simulink model "AircraftModel_6DoF"  (R2020b)
settings: Solver=VariableStepAuto  StartTime=0.0  StopTime=20  FixedStep=CNT_StepSize  RelTol=1e-3
values from neighbouring files (symbols this model uses):
  CNT_a = 6378137    [AircraftParameters.m]
  CNT_f = 0.003352810664747    (= 0.00335281066475)    [AircraftParameters.m]
  CNT_g = [0;0;9.81]    [AircraftParameters.m]
  CNT_m = 15917    [AircraftParameters.m]
  Ixx = 105390    [AircraftParameters.m]
  Ixz = 15539    [AircraftParameters.m]
  Iyy = 280790    [AircraftParameters.m]
  Izz = 350200    [AircraftParameters.m]
undefined symbols (not defined in the file or in its folder): Actuators, Aerodynamics, Propulsion, TrimPoint
libraries: vrlib x4
settings Model: Creator=NicolasS  LastModifiedBy=NicolasS

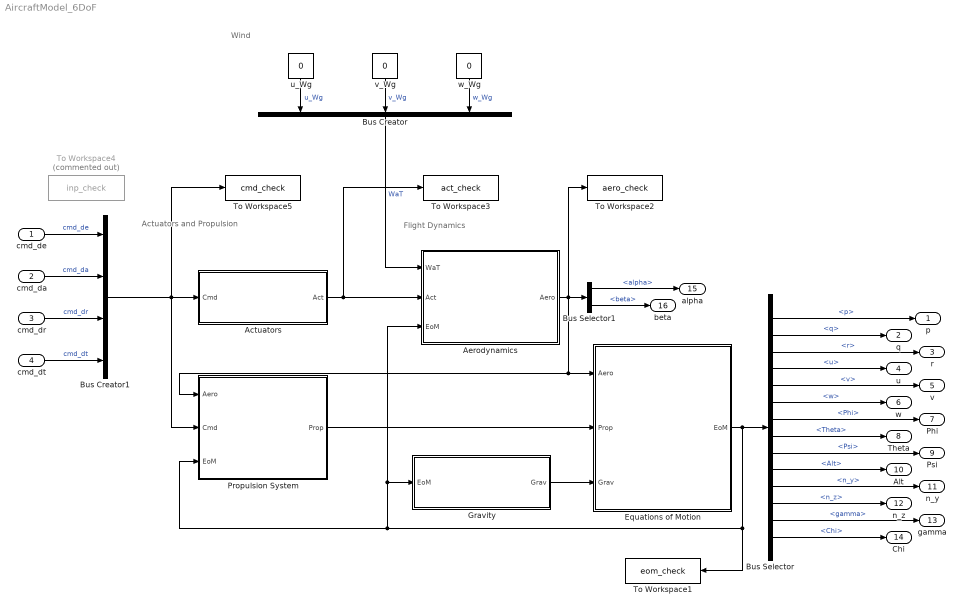
== system AircraftModel_6DoF ==
  note: Wind
  note: Actuators and Propulsion
  note: Flight Dynamics
  cmd_de : Inport
  cmd_da : Inport  Port=2
  cmd_dr : Inport  Port=3
  cmd_dt : Inport  Port=4
  Actuators : Subsystem
  Aerodynamics : Subsystem
  Bus Creator : BusCreator  Inputs=3
  Bus Creator1 : BusCreator  Inputs=4  OutDataTypeStr=Bus: Cmd
  Bus Selector : BusSelector  OutputSignals=OOmega_f.p,OOmega_f.q,OOmega_f.r,vv_f.u,vv_f.v,vv_f.w,PPhi.Phi,PPhi.Theta,PPhi.Psi,Position.Alt,nn_f.n_y,nn_f.n_z,TrackData.gamma,TrackData.Chi
  Bus Selector1 : BusSelector  OutputSignals=AirData.alpha,AirData.beta
  Equations of Motion : Subsystem
  Gravity : Subsystem
  "Propulsion System " : Subsystem
  To Workspace1 : ToWorkspace  VariableName=eom_check  SaveFormat=Timeseries  SampleTime=-1
      settings: Decimation=2
  To Workspace2 : ToWorkspace  VariableName=aero_check  SaveFormat=Timeseries  SampleTime=-1
      settings: Decimation=2
  To Workspace3 : ToWorkspace  VariableName=act_check  SaveFormat=Timeseries  SampleTime=-1
      settings: Decimation=2
  To Workspace4 : ToWorkspace  Commented=on  VariableName=inp_check  SaveFormat=Timeseries  SampleTime=-1
      settings: Decimation=2
  To Workspace5 : ToWorkspace  VariableName=cmd_check  SaveFormat=Timeseries  SampleTime=-1
      settings: Decimation=2
  u_Wg : Constant  Value=0  SampleTime=-1
  v_Wg : Constant  Value=0  SampleTime=-1
  w_Wg : Constant  Value=0  SampleTime=-1
  p : Outport  Unit=rad/s
  q : Outport  Port=2  Unit=rad/s
  r : Outport  Port=3  Unit=rad/s
  u : Outport  Port=4  Unit=m/s
  v : Outport  Port=5  Unit=m/s
  w : Outport  Port=6  Unit=m/s
  Phi : Outport  Port=7  Unit=rad
  Theta : Outport  Port=8  Unit=rad
  Psi : Outport  Port=9  Unit=rad
  Alt : Outport  Port=10  Unit=m
  n_y : Outport  Port=11
  n_z : Outport  Port=12
  gamma : Outport  Port=13  Unit=rad
  Chi : Outport  Port=14  Unit=rad
  alpha : Outport  Port=15
  beta : Outport  Port=16
  wires:
  u_Wg/1 -> Bus Creator/1  "u_Wg"
  Actuators/1(Act) -> To Workspace3/1, Aerodynamics/2(Act)
  Aerodynamics/1(Aero) -> To Workspace2/1, Bus Selector1/1, Equations of Motion/1(Aero), "Propulsion System "/1(Aero)
  w_Wg/1 -> Bus Creator/3  "w_Wg"
  Equations of Motion/1(EoM) -> To Workspace1/1, Aerodynamics/3(EoM), Gravity/1(EoM), "Propulsion System "/3(EoM), Bus Selector/1
  "Propulsion System "/1(Prop) -> Equations of Motion/2(Prop)
  Gravity/1(Grav) -> Equations of Motion/3(Grav)
  Bus Creator/1 -> Aerodynamics/1(WaT)  "WaT"
  Bus Selector1/2 -> beta/1  "<beta>"
  v_Wg/1 -> Bus Creator/2  "v_Wg"
  cmd_de/1 -> Bus Creator1/1  "cmd_de"
  cmd_dr/1 -> Bus Creator1/3  "cmd_dr"
  cmd_da/1 -> Bus Creator1/2  "cmd_da"
  cmd_dt/1 -> Bus Creator1/4  "cmd_dt"
  Bus Selector/3 -> r/1  "<r>"
  Bus Selector/9 -> Psi/1  "<Psi>"
  Bus Selector/7 -> Phi/1  "<Phi>"
  Bus Selector/1 -> p/1  "<p>"
  Bus Selector/11 -> n_y/1  "<n_y>"
  Bus Selector1/1 -> alpha/1  "<alpha>"
  Bus Selector/2 -> q/1  "<q>"
  Bus Selector/6 -> w/1  "<w>"
  Bus Selector/4 -> u/1  "<u>"
  Bus Selector/12 -> n_z/1  "<n_z>"
  Bus Selector/10 -> Alt/1  "<Alt>"
  Bus Selector/8 -> Theta/1  "<Theta>"
  Bus Creator1/1 -> To Workspace5/1, "Propulsion System "/2(Cmd), Actuators/1(Cmd)
  Bus Selector/13 -> gamma/1  "<gamma>"
  Bus Selector/14 -> Chi/1  "<Chi>"
  Bus Selector/5 -> v/1  "<v>"

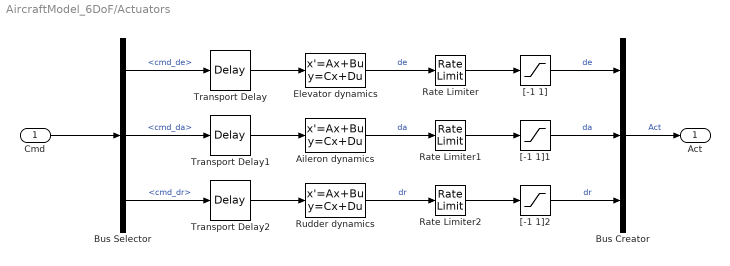
== system AircraftModel_6DoF/Actuators ==
  Cmd : Inport  OutDataTypeStr=Bus: Cmd
  Aileron dynamics : StateSpace  A=Actuators.Act_a.A  B=Actuators.Act_a.B  C=Actuators.Act_a.C  D=Actuators.Act_a.D  InitialCondition=TrimPoint.States.dabar  ContinuousStateAttributes='da'
  Bus Creator : BusCreator  Inputs=3  OutDataTypeStr=Bus: Act
  Bus Selector : BusSelector  OutputSignals=cmd_de,cmd_da,cmd_dr
  Elevator dynamics : StateSpace  A=Actuators.Act_e.A  B=Actuators.Act_e.B  C=Actuators.Act_e.C  D=Actuators.Act_e.D  InitialCondition=TrimPoint.States.debar  ContinuousStateAttributes='de'
  Rate Limiter : RateLimiter  RisingSlewLimit=max(Actuators.RateLimits.udot_max_He)  FallingSlewLimit=min(Actuators.RateLimits.udot_max_He)  SampleTimeMode=inherited
  Rate Limiter1 : RateLimiter  RisingSlewLimit=max(Actuators.RateLimits.udot_max_Ha)  FallingSlewLimit=min(Actuators.RateLimits.udot_max_Ha)  SampleTimeMode=inherited
  Rate Limiter2 : RateLimiter  RisingSlewLimit=max(Actuators.RateLimits.udot_max_Hr)  FallingSlewLimit=min(Actuators.RateLimits.udot_max_Hr)  SampleTimeMode=inherited
  Rudder dynamics : StateSpace  A=Actuators.Act_r.A  B=Actuators.Act_r.B  C=Actuators.Act_r.C  D=Actuators.Act_r.D  InitialCondition=TrimPoint.States.drbar  ContinuousStateAttributes='dr'
  Transport Delay : TransportDelay  DelayTime=Actuators.Delays.tau_de  InitialOutput=TrimPoint.States.debar  TransDelayFeedthrough=on
  Transport Delay1 : TransportDelay  DelayTime=Actuators.Delays.tau_da  InitialOutput=TrimPoint.States.dabar  TransDelayFeedthrough=on
  Transport Delay2 : TransportDelay  DelayTime=Actuators.Delays.tau_dr  InitialOutput=TrimPoint.States.drbar  TransDelayFeedthrough=on
  "[-1 1]" : Saturate  UpperLimit=max(Actuators.Limits.u_max_He)  LowerLimit=min(Actuators.Limits.u_max_He)
  "[-1 1]1" : Saturate  UpperLimit=max(Actuators.Limits.u_max_Ha)  LowerLimit=min(Actuators.Limits.u_max_Ha)
  "[-1 1]2" : Saturate  UpperLimit=max(Actuators.Limits.u_max_Hr)  LowerLimit=min(Actuators.Limits.u_max_Hr)
  Act : Outport  OutDataTypeStr=Bus: Act
  wires:
  Elevator dynamics/1 -> Rate Limiter/1  "de"
  "[-1 1]1"/1 -> Bus Creator/2  "da"
  Rudder dynamics/1 -> Rate Limiter2/1  "dr"
  Transport Delay1/1 -> Aileron dynamics/1
  Cmd/1 -> Bus Selector/1
  "[-1 1]"/1 -> Bus Creator/1  "de"
  Bus Selector/1 -> Transport Delay/1  "<cmd_de>"
  Transport Delay/1 -> Elevator dynamics/1
  "[-1 1]2"/1 -> Bus Creator/3  "dr"
  Transport Delay2/1 -> Rudder dynamics/1
  Aileron dynamics/1 -> Rate Limiter1/1  "da"
  Bus Selector/3 -> Transport Delay2/1  "<cmd_dr>"
  Bus Creator/1 -> Act/1  "Act"
  Bus Selector/2 -> Transport Delay1/1  "<cmd_da>"
  Rate Limiter/1 -> "[-1 1]"/1
  Rate Limiter1/1 -> "[-1 1]1"/1
  Rate Limiter2/1 -> "[-1 1]2"/1

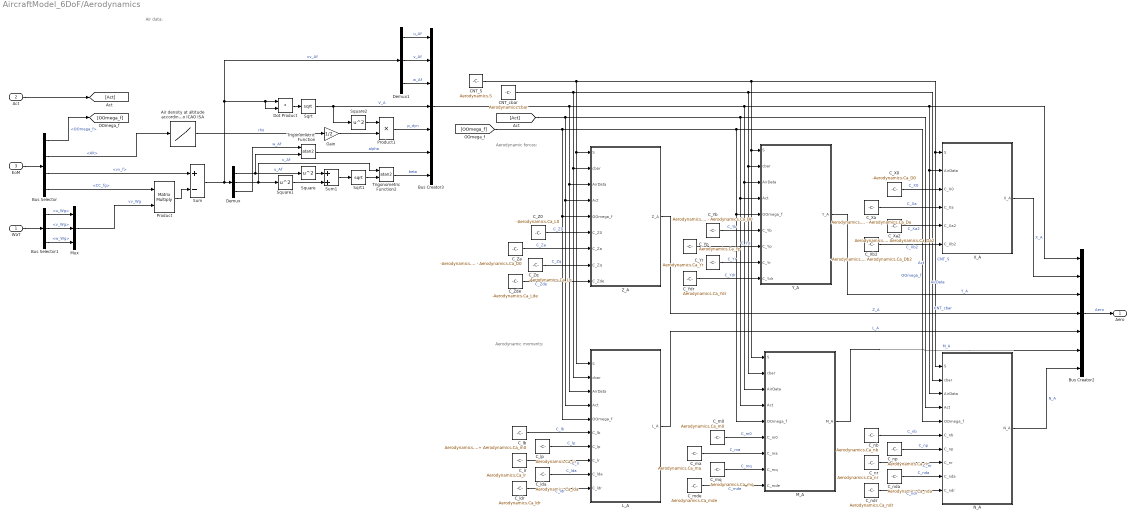
== system AircraftModel_6DoF/Aerodynamics ==
  note: Air data:
  note: Aerodynamic moments:
  note: Aerodynamic forces:
  WaT : Inport  OutDataTypeStr=Bus: WaT
  Act : Inport  Port=2  OutDataTypeStr=Bus: Act
  EoM : Inport  Port=3  OutDataTypeStr=Bus: EoM
  Air density at altitude according to ICAO ISA : Lookup_n-D  NumberOfTableDimensions=1  BreakpointsForDimension1=Aerodynamics.LUT_Alt  Table=Aerodynamics.LUT_rho  ExtrapMethod=Clip  InternalRulePriority=Speed  RndMeth=Simplest  InputSameDT=on
  Bus Creator2 : BusCreator  Inputs=7  OutDataTypeStr=Bus: Aero
  Bus Creator3 : BusCreator  Inputs=7  OutDataTypeStr=Bus: AirData
  Bus Selector : BusSelector  OutputSignals=OOmega_f,Position.Alt,vv_f,CC.CC_fg
  Bus Selector1 : BusSelector  OutputSignals=u_Wg,v_Wg,w_Wg
  CNT_S : Constant  Value=Aerodynamics.S  OutDataTypeStr=double  SampleTime=-1
  CNT_cbar : Constant  Value=Aerodynamics.cbar  OutDataTypeStr=double  SampleTime=-1
  C_X0 : Constant  Value=-Aerodynamics.Ca_D0  VectorParams1D=off  OutDataTypeStr=double  SampleTime=-1
  C_Xa : Constant  Value=Aerodynamics.Ca_L0 - Aerodynamics.Ca_Da  VectorParams1D=off  OutDataTypeStr=double  SampleTime=-1
  C_Xa2 : Constant  Value=Aerodynamics.Ca_La - Aerodynamics.Ca_Da2  VectorParams1D=off  OutDataTypeStr=double  SampleTime=-1
  C_Xb2 : Constant  Value=-Aerodynamics.Ca_Yb - Aerodynamics.Ca_Db2  VectorParams1D=off  OutDataTypeStr=double  SampleTime=-1
  C_Yb : Constant  Value=Aerodynamics.Ca_Yb - Aerodynamics.Ca_D0  VectorParams1D=off  OutDataTypeStr=double  SampleTime=-1
  C_Ydr : Constant  Value=Aerodynamics.Ca_Ydr  VectorParams1D=off  OutDataTypeStr=double  SampleTime=-1
  C_Yp : Constant  Value=Aerodynamics.Ca_Yp  VectorParams1D=off  OutDataTypeStr=double  SampleTime=-1
  C_Yr : Constant  Value=Aerodynamics.Ca_Yr  VectorParams1D=off  OutDataTypeStr=double  SampleTime=-1
  C_Z0 : Constant  Value=-Aerodynamics.Ca_L0  VectorParams1D=off  OutDataTypeStr=double  SampleTime=-1
  C_Za : Constant  Value=-Aerodynamics.Ca_La - Aerodynamics.Ca_D0  VectorParams1D=off  OutDataTypeStr=double  SampleTime=-1
  C_Zde : Constant  Value=-Aerodynamics.Ca_Lde  VectorParams1D=off  OutDataTypeStr=double  SampleTime=-1
  C_Zq : Constant  Value=-Aerodynamics.Ca_Lq  VectorParams1D=off  OutDataTypeStr=double  SampleTime=-1
  C_lb : Constant  Value=Aerodynamics.Ca_lb + Aerodynamics.Ca_m0  VectorParams1D=off  OutDataTypeStr=double  SampleTime=-1
  C_lda : Constant  Value=Aerodynamics.Ca_lda  VectorParams1D=off  OutDataTypeStr=double  SampleTime=-1
  C_ldr : Constant  Value=Aerodynamics.Ca_ldr  VectorParams1D=off  OutDataTypeStr=double  SampleTime=-1
  C_lp : Constant  Value=Aerodynamics.Ca_lp  VectorParams1D=off  OutDataTypeStr=double  SampleTime=-1
  C_lr : Constant  Value=Aerodynamics.Ca_lr  VectorParams1D=off  OutDataTypeStr=double  SampleTime=-1
  C_m0 : Constant  Value=Aerodynamics.Ca_m0  VectorParams1D=off  OutDataTypeStr=double  SampleTime=-1
  C_ma : Constant  Value=Aerodynamics.Ca_ma  VectorParams1D=off  OutDataTypeStr=double  SampleTime=-1
  C_mde : Constant  Value=Aerodynamics.Ca_mde  VectorParams1D=off  OutDataTypeStr=double  SampleTime=-1
  C_mq : Constant  Value=Aerodynamics.Ca_mq  VectorParams1D=off  OutDataTypeStr=double  SampleTime=-1
  C_nb : Constant  Value=Aerodynamics.Ca_nb  VectorParams1D=off  OutDataTypeStr=double  SampleTime=-1
  C_nda : Constant  Value=Aerodynamics.Ca_nda  VectorParams1D=off  OutDataTypeStr=double  SampleTime=-1
  C_ndr : Constant  Value=Aerodynamics.Ca_ndr  VectorParams1D=off  OutDataTypeStr=double  SampleTime=-1
  C_np : Constant  Value=Aerodynamics.Ca_np  VectorParams1D=off  OutDataTypeStr=double  SampleTime=-1
  C_nr : Constant  Value=Aerodynamics.Ca_nr  VectorParams1D=off  OutDataTypeStr=double  SampleTime=-1
  Demux : Demux  Outputs=3
  Demux1 : Demux  Outputs=3
  Dot Product : DotProduct  InputSameDT=on  OutDataTypeStr=Inherit: Inherit via internal rule
  Gain : Gain  Gain=1/2
  L_A : MATLAB Function  TreatAsAtomicUnit=on
  M_A : MATLAB Function  TreatAsAtomicUnit=on
  Mux : Mux  Inputs=3
  N_A : MATLAB Function  TreatAsAtomicUnit=on
  Product : Product  Multiplication=Matrix(*)
  Product1 : Product
  Sqrt : Sqrt  SaturateOnIntegerOverflow=on
  Sqrt1 : Sqrt  SaturateOnIntegerOverflow=on
  Square : Math  Operator=square  SaturateOnIntegerOverflow=on
  Square1 : Math  Operator=square  SaturateOnIntegerOverflow=on
  Square2 : Math  Operator=square  SaturateOnIntegerOverflow=on
  Sum : Sum  Inputs=+-
  Sum1 : Sum
  Trigonometric Function : Trigonometry  Operator=atan2
  Trigonometric Function2 : Trigonometry  Operator=atan2
  X_A : MATLAB Function  TreatAsAtomicUnit=on
  Y_A : MATLAB Function  TreatAsAtomicUnit=on
  Z_A : MATLAB Function  TreatAsAtomicUnit=on
  Aero : Outport  OutDataTypeStr=Bus: Aero
  wires:
  Demux1/3 -> Bus Creator3/3  "w_Af"
  C_lp/1 -> L_A/7(C_lp)  "C_lp"
  Act/1 -> [Act]
  N_A/1(N_A) -> Bus Creator2/7  "N_A"
  C_nb/1 -> N_A/6(C_nb)  "C_nb"
  C_ldr/1 -> L_A/10(C_ldr)  "C_ldr"
  C_m0/1 -> M_A/6(C_m0)  "C_m0"
  C_Zq/1 -> Z_A/8(C_Zq)  "C_Zq"
  [OOmega_f] -> N_A/5(OOmega_f), M_A/5(OOmega_f), Y_A/5(OOmega_f), L_A/5(OOmega_f), Z_A/5(OOmega_f)  "OOmega_f"
  C_lr/1 -> L_A/8(C_lr)  "C_lr"
  C_mq/1 -> M_A/8(C_mq)  "C_mq"
  Air density at altitude according to ICAO ISA/1 -> Gain/1  "rho"
  C_Z0/1 -> Z_A/6(C_Z0)  "C_Z0"
  Square/1 -> Sum1/1
  X_A/1(X_A) -> Bus Creator2/2  "X_A"
  Trigonometric Function2/1 -> Bus Creator3/7  "beta"
  C_Yr/1 -> Y_A/8(C_Yr)  "C_Yr"
  C_Yb/1 -> Y_A/6(C_Yb)  "C_Yb"
  Demux1/2 -> Bus Creator3/2  "v_Af"
  Dot Product/1 -> Sqrt/1
  C_ma/1 -> M_A/7(C_ma)  "C_ma"
  C_nda/1 -> N_A/9(C_nda)  "C_nda"
  C_Xa/1 -> X_A/4(C_Xa)  "C_Xa"
  C_lb/1 -> L_A/6(C_lb)  "C_lb"
  Sum/1 -> Demux/1, Demux1/1, Dot Product/2, Dot Product/1  "vv_Af"
  C_Xa2/1 -> X_A/5(C_Xa2)  "C_Xa2"
  C_Ydr/1 -> Y_A/9(C_Ydr)  "C_Ydr"
  C_Xb2/1 -> X_A/6(C_Xb2)  "C_Xb2"
  Y_A/1(Y_A) -> Bus Creator2/3  "Y_A"
  C_Za/1 -> Z_A/7(C_Za)  "C_Za"
  CNT_S/1 -> N_A/1(S), X_A/1(S), M_A/1(S), Y_A/1(S), L_A/1(S), Z_A/1(S)  "CNT_S"
  C_nr/1 -> N_A/8(C_nr)  "C_nr"
  Bus Creator2/1 -> Aero/1  "Aero"
  C_mde/1 -> M_A/9(C_mde)  "C_mde"
  [Act] -> N_A/4(Act), M_A/4(Act), Y_A/4(Act), L_A/4(Act), Z_A/4(Act)  "Act"
  Demux/3 -> Trigonometric Function/1  "w_Af"
  C_X0/1 -> X_A/3(C_X0)  "C_X0"
  C_np/1 -> N_A/7(C_np)  "C_np"
  Demux/2 -> Square1/1, Trigonometric Function2/1  "v_Af"
  C_Yp/1 -> Y_A/7(C_Yp)  "C_Yp"
  C_ndr/1 -> N_A/10(C_ndr)  "C_ndr"
  Demux/1 -> Square/1, Trigonometric Function/2  "u_Af"
  Bus Creator3/1 -> L_A/3(AirData), Z_A/3(AirData), Bus Creator2/1, N_A/3(AirData), X_A/2(AirData), M_A/3(AirData), Y_A/3(AirData)  "AirData"
  M_A/1(M_A) -> Bus Creator2/6  "M_A"
  Sqrt1/1 -> Trigonometric Function2/2
  Bus Selector/2 -> Air density at altitude according to ICAO ISA/1  "<Alt>"
  C_Zde/1 -> Z_A/9(C_Zde)  "C_Zde"
  Gain/1 -> Product1/2
  Product/1 -> Sum/2
  C_lda/1 -> L_A/9(C_lda)  "C_lda"
  L_A/1(L_A) -> Bus Creator2/5  "L_A"
  Demux1/1 -> Bus Creator3/1  "u_Af"
  Z_A/1(Z_A) -> Bus Creator2/4  "Z_A"
  Product1/1 -> Bus Creator3/5  "p_dyn"
  Sqrt/1 -> Square2/1, Bus Creator3/4  "V_A"
  CNT_cbar/1 -> N_A/2(cbar), M_A/2(cbar), Y_A/2(cbar), L_A/2(cbar), Z_A/2(cbar)  "CNT_cbar"
  Trigonometric Function/1 -> Bus Creator3/6  "alpha"
  Bus Selector/3 -> Sum/1  "<vv_f>"
  Sum1/1 -> Sqrt1/1
  EoM/1 -> Bus Selector/1
  Bus Selector/1 -> [OOmega_f]  "<OOmega_f>"
  Bus Selector/4 -> Product/1  "<CC_fg>"
  Square2/1 -> Product1/1
  Square1/1 -> Sum1/2
  WaT/1 -> Bus Selector1/1
  Bus Selector1/1 -> Mux/1  "<u_Wg>"
  Bus Selector1/2 -> Mux/2  "<v_Wg>"
  Bus Selector1/3 -> Mux/3  "<w_Wg>"
  Mux/1 -> Product/2  "vv_Wg"

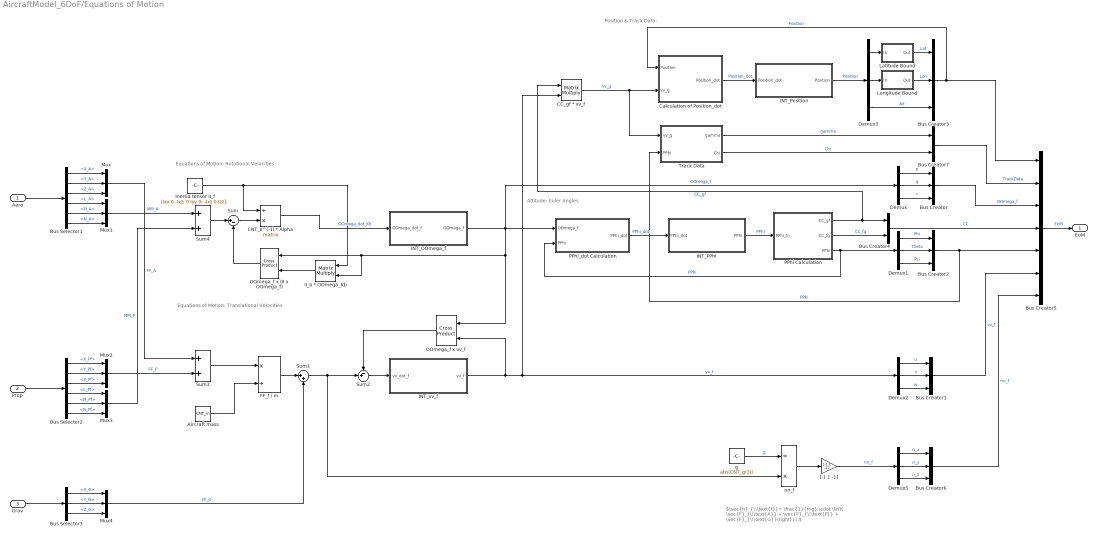
== system AircraftModel_6DoF/Equations of Motion ==
  note: Equations of Motion: Translational Velocities
  note: Equations of Motion: Rotational Velocities
  note: Attitude: Euler Angles
  note: Position & Track Data:
  note: $\vec{n}_{\!\text{f}}= \frac{1}{mg} \cdot \left( \vec{F}_{\!\text{A}} + \vec{F}_{\!\text{P}} + \vec{F}_{\!\text{G}}\right) \,\,$
  Aero : Inport  OutDataTypeStr=Bus: Aero
  Prop : Inport  Port=2  OutDataTypeStr=Bus: Prop
  Grav : Inport  Port=3  OutDataTypeStr=Bus: Grav
  Aircraft mass : Constant  Value=CNT_m  SampleTime=-1
  Bus Creator : BusCreator  Inputs=3  OutDataTypeStr=Bus: OOmega_f
  Bus Creator1 : BusCreator  Inputs=3  OutDataTypeStr=Bus: vv_f
  Bus Creator2 : BusCreator  Inputs=3  OutDataTypeStr=Bus: PPhi
  Bus Creator3 : BusCreator  Inputs=3  OutDataTypeStr=Bus: Position
  Bus Creator4 : BusCreator  Inputs=2  OutDataTypeStr=Bus: CC
  Bus Creator5 : BusCreator  Inputs=7  OutDataTypeStr=Bus: EoM
  Bus Creator6 : BusCreator  Inputs=3  OutDataTypeStr=Bus: nn_f
  Bus Creator7 : BusCreator  Inputs=2  OutDataTypeStr=Bus: TrackData
  Bus Selector1 : BusSelector  OutputSignals=X_A,Y_A,Z_A,L_A,M_A,N_A
  Bus Selector2 : BusSelector  OutputSignals=X_Pf,Y_Pf,Z_Pf,L_Pf,M_Pf,N_Pf
  Bus Selector3 : BusSelector  OutputSignals=X_G,Y_G,Z_G
  CC_gf * vv_f : Product  Multiplication=Matrix(*)  RndMeth=Zero
  CNT_II^(-1) * Alpha : Product  Inputs=/*  Multiplication=Matrix(*)
  Calculation of Position_dot : Subsystem
  Demux{,1..3,5} (5 alike) : Demux  Outputs=3
  FF_f / m : Product  Inputs=*/
  II_b * OOmega_Kb : Product  Multiplication=Matrix(*)  RndMeth=Zero
  INT_OOmega_f : Subsystem
  INT_PPhi : Subsystem
  INT_Position : Subsystem
  INT_vv_f : Subsystem
  Inertia tensor II_f : Constant  Value=[Ixx 0 -Ixz; 0 Iyy 0; -Ixz 0 Izz];  SampleTime=-1
  Latitude Bound : Subsystem  mask(Latitude bound){}
      mask help: Bounds the latitude to [-pi/2, pi/2]. When the lower bound is exceeded the latitude is increasing again; when the upper bound is exceeded the latitude is decreasing.
  Longitude Bound : Subsystem  mask(Longitude bound){}
      mask help: Bounds the longitude to [-pi, pi]. When -pi bound is exceeded the longitude wraps back to pi; when the pi bound is exceeded the longitude wraps back to -pi.
  Mux{,1..4} (5 alike) : Mux  Inputs=3
  OOmega_f x (II x OOmega_f) : vrlib/Utilities/Cross Product
  OOmega_f x vv_f : vrlib/Utilities/Cross Product
  PPhi Calculation : MATLAB Function  TreatAsAtomicUnit=on
  PPhi_dot Calculation : MATLAB Function  TreatAsAtomicUnit=on
  Sum : Sum  Inputs=|+-
  Sum1 : Sum  Inputs=|++
  Sum2 : Sum  Inputs=-+|
  Sum3 : Sum
  Sum4 : Sum
  Track Data : Subsystem
  "[-1 1 -1]" : Gain  Gain=[-1 1 -1]'
  g : Constant  Value=abs(CNT_g(3))  SampleTime=-1
  "nn_f " : Product  Inputs=/*  RndMeth=Zero
  EoM : Outport  OutDataTypeStr=Bus: EoM
  wires:
  Longitude Bound/1(Out) -> Bus Creator3/2  "Lon"
  "[-1 1 -1]"/1 -> Demux5/1  "nn_f"
  Bus Selector1/6 -> Mux1/3  "<N_A>"
  Bus Creator/1 -> Bus Creator5/3  "OOmega_f"
  Bus Selector2/5 -> Mux3/2  "<M_Pf>"
  INT_OOmega_f/1(OOmega_f) -> Demux/1, II_b * OOmega_Kb/2, OOmega_f x (II x OOmega_f)/1, OOmega_f x vv_f/1, PPhi_dot Calculation/1(OOmega_f)  "OOmega_f"
  Demux/2 -> Bus Creator/2  "q"
  Prop/1 -> Bus Selector2/1
  Mux1/1 -> Sum4/1  "MM_A"
  Demux/1 -> Bus Creator/1  "p"
  Demux1/2 -> Bus Creator2/2  "Theta"
  Bus Creator1/1 -> Bus Creator5/6  "vv_f"
  Demux3/2 -> Longitude Bound/1(In)
  INT_vv_f/1(vv_f) -> Demux2/1, CC_gf * vv_f/2, OOmega_f x vv_f/2  "vv_f"
  Mux2/1 -> Sum3/2  "FF_P"
  "nn_f "/1 -> "[-1 1 -1]"/1
  Demux2/3 -> Bus Creator1/3  "w"
  Bus Selector2/3 -> Mux2/3  "<Z_Pf>"
  Demux5/1 -> Bus Creator6/1  "n_x"
  Bus Creator6/1 -> Bus Creator5/7  "nn_f"
  Demux5/2 -> Bus Creator6/2  "n_y"
  Demux/3 -> Bus Creator/3  "r"
  OOmega_f x vv_f/1 -> Sum2/1
  Bus Selector2/2 -> Mux2/2  "<Y_Pf>"
  g/1 -> "nn_f "/1  "g"
  Bus Selector1/3 -> Mux/3  "<Z_A>"
  Mux/1 -> Sum3/1  "FF_A"
  PPhi Calculation/1(CC_gf) -> CC_gf * vv_f/1, Bus Creator4/1  "CC_gf"
  Bus Selector1/4 -> Mux1/1  "<L_A>"
  INT_PPhi/1(PPhi) -> PPhi Calculation/1(PPhi_In)  "PPhi"
  PPhi Calculation/3(PPhi) -> PPhi_dot Calculation/2(PPhi), Demux1/1  "PPhi"
  Bus Creator3/1 -> Bus Creator5/1, Calculation of Position_dot/1(Position)  "Position"
  CC_gf * vv_f/1 -> Track Data/1(vv_g), Calculation of Position_dot/2(vv_g)  "vv_g"
  Mux3/1 -> Sum4/2  "MM_P"
  Aircraft mass/1 -> FF_f / m/2
  PPhi Calculation/2(CC_fg) -> Bus Creator4/2  "CC_fg"
  Aero/1 -> Bus Selector1/1
  Calculation of Position_dot/1(Position_dot) -> INT_Position/1(Position_dot)  "Position_dot"
  Demux3/3 -> Bus Creator3/3  "Alt"
  Sum3/1 -> FF_f / m/1
  Bus Selector1/2 -> Mux/2  "<Y_A>"
  Demux2/1 -> Bus Creator1/1  "u"
  Sum2/1 -> INT_vv_f/1(vv_dot_f)
  Demux2/2 -> Bus Creator1/2  "v"
  PPhi_dot Calculation/1(PPhi_dot) -> INT_PPhi/1(PPhi_dot)  "PPhi_dot"
  Bus Creator2/1 -> Track Data/2(PPhi), Bus Creator5/5  "PPhi"
  Bus Creator4/1 -> Bus Creator5/4  "CC"
  OOmega_f x (II x OOmega_f)/1 -> Sum/2
  Latitude Bound/1(Out) -> Bus Creator3/1  "Lat"
  Sum1/1 -> "nn_f "/2, Sum2/2
  FF_f / m/1 -> Sum1/1
  II_b * OOmega_Kb/1 -> OOmega_f x (II x OOmega_f)/2
  Bus Selector1/5 -> Mux1/2  "<M_A>"
  Demux1/1 -> Bus Creator2/1  "Phi"
  Bus Selector2/1 -> Mux2/1  "<X_Pf>"
  Sum/1 -> CNT_II^(-1) * Alpha/2
  Demux3/1 -> Latitude Bound/1(In)
  Bus Selector2/4 -> Mux3/1  "<L_Pf>"
  Demux1/3 -> Bus Creator2/3  "Psi"
  INT_Position/1(Position) -> Demux3/1  "Position"
  Inertia tensor II_f/1 -> CNT_II^(-1) * Alpha/1, II_b * OOmega_Kb/1
  Bus Selector1/1 -> Mux/1  "<X_A>"
  CNT_II^(-1) * Alpha/1 -> INT_OOmega_f/1(OOmega_dot_f)  "OOmega_dot_Kb"
  Bus Selector2/6 -> Mux3/3  "<N_Pf>"
  Sum4/1 -> Sum/1
  Demux5/3 -> Bus Creator6/3  "n_z"
  Bus Creator5/1 -> EoM/1  "EoM"
  Mux4/1 -> Sum1/2  "FF_G"
  Bus Selector3/1 -> Mux4/1  "<X_G>"
  Grav/1 -> Bus Selector3/1
  Bus Selector3/2 -> Mux4/2  "<Y_G>"
  Bus Selector3/3 -> Mux4/3  "<Z_G>"
  Track Data/1(gamma) -> Bus Creator7/1  "gamma"
  Track Data/2(Chi) -> Bus Creator7/2  "Chi"
  Bus Creator7/1 -> Bus Creator5/2  "TrackData"

== system AircraftModel_6DoF/Gravity ==
  note: Gravitational Force
  EoM : Inport  OutDataTypeStr=Bus: EoM
  Bus Creator : BusCreator  Inputs=3  OutDataTypeStr=Bus: Grav
  Bus Selector : BusSelector  OutputSignals=CC.CC_fg
  CC_fg * gg : Product  Multiplication=Matrix(*)  RndMeth=Zero
  Demux : Demux  Outputs=3
  Grav. Acc. : Constant  Value=CNT_g  SampleTime=-1
  Grav : Outport  OutDataTypeStr=Bus: Grav
  wires:
  EoM/1 -> Bus Selector/1
  Bus Selector/1 -> CC_fg * gg/1  "<CC_fg>"
  CC_fg * gg/1 -> Demux/1  "gg_f"
  Grav. Acc./1 -> CC_fg * gg/2  "gg"
  Demux/1 -> Bus Creator/1  "X_G"
  Demux/2 -> Bus Creator/2  "Y_G"
  Demux/3 -> Bus Creator/3  "Z_G"
  Bus Creator/1 -> Grav/1

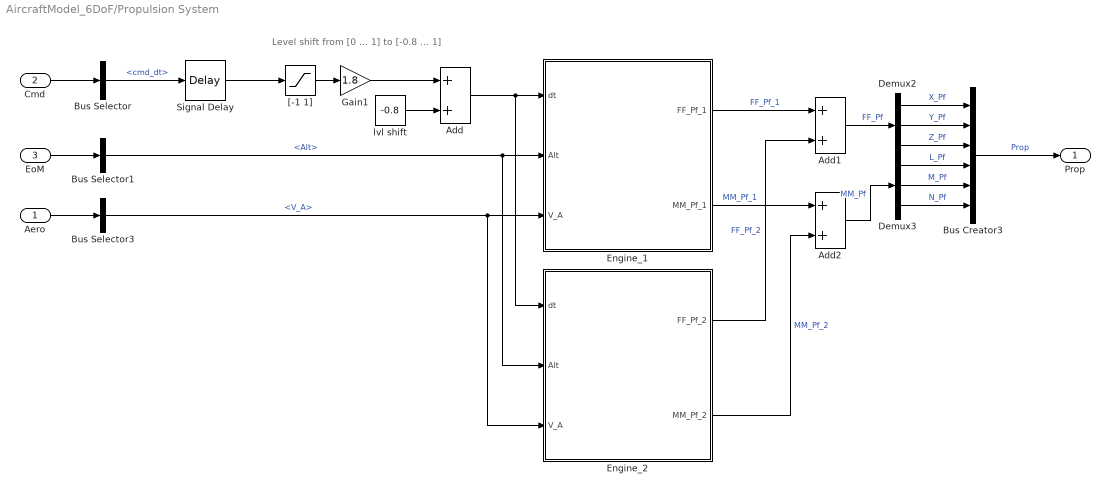
== system AircraftModel_6DoF/Propulsion System  ==
  note: Level shift from [0 ... 1] to [-0.8 ... 1]
  Aero : Inport  OutDataTypeStr=Bus: Aero
  Cmd : Inport  Port=2  OutDataTypeStr=Bus: Cmd
  EoM : Inport  Port=3  OutDataTypeStr=Bus: EoM
  Add : Sum
  Add1 : Sum
  Add2 : Sum
  Bus Creator3 : BusCreator  Inputs=6  OutDataTypeStr=Bus: Prop
  Bus Selector : BusSelector  OutputSignals=cmd_dt
  Bus Selector1 : BusSelector  OutputSignals=Position.Alt
  Bus Selector3 : BusSelector  OutputSignals=AirData.V_A
  Demux2 : Demux  Outputs=3
  Demux3 : Demux  Outputs=3
  Engine_1 : Subsystem
  Engine_2 : Subsystem
  Gain1 : Gain  Gain=1.8
  Signal Delay : TransportDelay  DelayTime=Propulsion.Delays.tau_dt  InitialOutput=TrimPoint.States.dtbar  TransDelayFeedthrough=on
  "[-1 1]" : Saturate  UpperLimit=1  LowerLimit=0
  lvl shift : Constant  Value=-0.8  SampleTime=-1
  Prop : Outport  OutDataTypeStr=Bus: Prop
  wires:
  Demux2/2 -> Bus Creator3/2  "Y_Pf"
  Engine_1/1(FF_Pf_1) -> Add1/1  "FF_Pf_1"
  Demux3/1 -> Bus Creator3/4  "L_Pf"
  EoM/1 -> Bus Selector1/1
  lvl shift/1 -> Add/2
  Engine_2/1(FF_Pf_2) -> Add1/2  "FF_Pf_2"
  Add2/1 -> Demux3/1  "MM_Pf"
  Bus Selector3/1 -> Engine_2/3(V_A), Engine_1/3(V_A)  "<V_A>"
  Aero/1 -> Bus Selector3/1
  Demux2/1 -> Bus Creator3/1  "X_Pf"
  Gain1/1 -> Add/1
  Engine_1/2(MM_Pf_1) -> Add2/1  "MM_Pf_1"
  Add/1 -> Engine_2/1(dt), Engine_1/1(dt)
  Bus Creator3/1 -> Prop/1  "Prop"
  Demux3/2 -> Bus Creator3/5  "M_Pf"
  "[-1 1]"/1 -> Gain1/1
  Demux2/3 -> Bus Creator3/3  "Z_Pf"
  Add1/1 -> Demux2/1  "FF_Pf"
  Bus Selector1/1 -> Engine_2/2(Alt), Engine_1/2(Alt)  "<Alt>"
  Demux3/3 -> Bus Creator3/6  "N_Pf"
  Cmd/1 -> Bus Selector/1
  Bus Selector/1 -> Signal Delay/1  "<cmd_dt>"
  Engine_2/2(MM_Pf_2) -> Add2/2  "MM_Pf_2"
  Signal Delay/1 -> "[-1 1]"/1

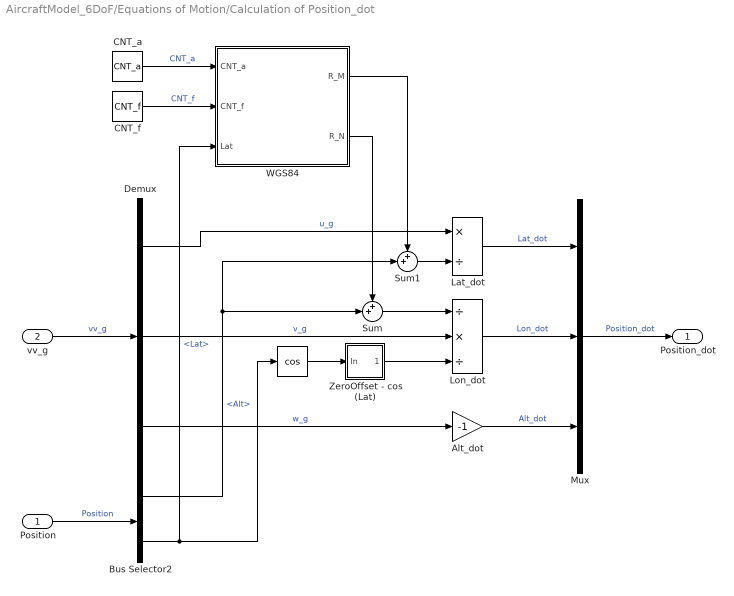
== system AircraftModel_6DoF/Equations of Motion/Calculation of Position_dot ==
  Position : Inport  OutDataTypeStr=Bus: Position
  vv_g : Inport  Port=2
  " " : Trigonometry  Operator=cos
  Alt_dot : Gain  Gain=-1
  Bus Selector2 : BusSelector  OutputSignals=Alt,Lat
  CNT_a : Constant  Value=CNT_a  SampleTime=-1
  CNT_f : Constant  Value=CNT_f  SampleTime=-1
  Demux : Demux  Outputs=3
  Lat_dot : Product  Inputs=*/
  Lon_dot : Product  Inputs=/*/
  Mux : Mux  Inputs=3
  Sum : Sum  Inputs=++|
  Sum1 : Sum  Inputs=++|
  WGS84 : MATLAB Function  TreatAsAtomicUnit=on
  ZeroOffset - cos (Lat) : Subsystem  mask(Zero offset){tol=1E-5}
      mask prompts: tol "Tolerance"
      mask help: This block outputs a value equal to the tolerance specified in the block parameters if the input falls within a sphere with this tolerance as radius and center in the origin. Otherwise, the output equals the input.
      mask Help: This block outputs a value equal to the tolerance specified in the block parameters if the input falls within a sphere with this tolerance as radius and center in the origin. Otherwise, the output equals the input.
  Position_dot : Outport
  wires:
  ZeroOffset - cos (Lat)/1(Out) -> Lon_dot/3
  Mux/1 -> Position_dot/1  "Position_dot"
  vv_g/1 -> Demux/1  "vv_g"
  Position/1 -> Bus Selector2/1  "Position"
  Lat_dot/1 -> Mux/1  "Lat_dot"
  Lon_dot/1 -> Mux/2  "Lon_dot"
  Alt_dot/1 -> Mux/3  "Alt_dot"
  Demux/3 -> Alt_dot/1  "w_g"
  Demux/1 -> Lat_dot/1  "u_g"
  Demux/2 -> Lon_dot/2  "v_g"
  Sum/1 -> Lon_dot/1
  Sum1/1 -> Lat_dot/2
  WGS84/2(R_N) -> Sum/1
  WGS84/1(R_M) -> Sum1/1
  Bus Selector2/1 -> Sum1/2, Sum/2  "<Alt>"
  " "/1 -> ZeroOffset - cos (Lat)/1(In)
  Bus Selector2/2 -> WGS84/3(Lat), " "/1  "<Lat>"
  CNT_a/1 -> WGS84/1(CNT_a)  "CNT_a"
  CNT_f/1 -> WGS84/2(CNT_f)  "CNT_f"

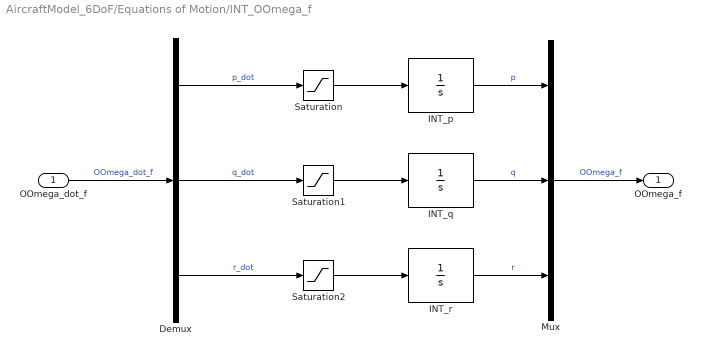
== system AircraftModel_6DoF/Equations of Motion/INT_OOmega_f ==
  OOmega_dot_f : Inport
  Demux : Demux  Outputs=3
  INT_p : Integrator  InitialCondition=TrimPoint.States.pbar  ContinuousStateAttributes='p'
  INT_q : Integrator  InitialCondition=TrimPoint.States.qbar  ContinuousStateAttributes='q'
  INT_r : Integrator  InitialCondition=TrimPoint.States.rbar  ContinuousStateAttributes='r'
  Mux : Mux  Inputs=3
  Saturation : Saturate  UpperLimit=100000  LowerLimit=-100000
  Saturation1 : Saturate  UpperLimit=100000  LowerLimit=-100000
  Saturation2 : Saturate  UpperLimit=100000  LowerLimit=-100000
  OOmega_f : Outport
  wires:
  Mux/1 -> OOmega_f/1  "OOmega_f"
  INT_r/1 -> Mux/3  "r"
  INT_q/1 -> Mux/2  "q"
  INT_p/1 -> Mux/1  "p"
  Demux/3 -> Saturation2/1  "r_dot"
  Demux/2 -> Saturation1/1  "q_dot"
  Demux/1 -> Saturation/1  "p_dot"
  OOmega_dot_f/1 -> Demux/1  "OOmega_dot_f"
  Saturation/1 -> INT_p/1
  Saturation1/1 -> INT_q/1
  Saturation2/1 -> INT_r/1

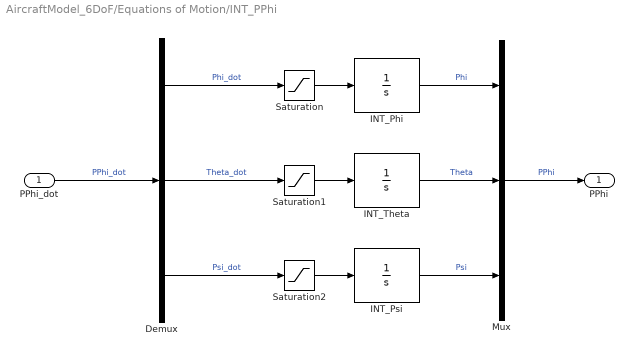
== system AircraftModel_6DoF/Equations of Motion/INT_PPhi ==
  PPhi_dot : Inport
  Demux : Demux  Outputs=3
  INT_Phi : Integrator  InitialCondition=TrimPoint.States.Phibar  ContinuousStateAttributes='Phi'
  INT_Psi : Integrator  InitialCondition=TrimPoint.States.Psibar  ContinuousStateAttributes='Psi'
  INT_Theta : Integrator  InitialCondition=TrimPoint.States.Thetabar  ContinuousStateAttributes='Theta'
  Mux : Mux  Inputs=3
  Saturation : Saturate  UpperLimit=100000  LowerLimit=-100000
  Saturation1 : Saturate  UpperLimit=100000  LowerLimit=-100000
  Saturation2 : Saturate  UpperLimit=100000  LowerLimit=-100000
  PPhi : Outport
  wires:
  Saturation2/1 -> INT_Psi/1
  Saturation1/1 -> INT_Theta/1
  Saturation/1 -> INT_Phi/1
  Mux/1 -> PPhi/1  "PPhi"
  INT_Psi/1 -> Mux/3  "Psi"
  INT_Theta/1 -> Mux/2  "Theta"
  INT_Phi/1 -> Mux/1  "Phi"
  Demux/3 -> Saturation2/1  "Psi_dot"
  Demux/2 -> Saturation1/1  "Theta_dot"
  Demux/1 -> Saturation/1  "Phi_dot"
  PPhi_dot/1 -> Demux/1  "PPhi_dot"

== system AircraftModel_6DoF/Equations of Motion/INT_Position ==
  Position_dot : Inport
  Demux : Demux  Outputs=3
  INT_Alt : Integrator  InitialCondition=TrimPoint.States.Altbar  ContinuousStateAttributes='Alt'
  INT_Lat : Integrator  InitialCondition=TrimPoint.States.Latbar  ContinuousStateAttributes='Lat'
  INT_Lon : Integrator  InitialCondition=TrimPoint.States.Lonbar  ContinuousStateAttributes='Lon'
  Mux : Mux  Inputs=3
  Saturation : Saturate  UpperLimit=100000  LowerLimit=-100000
  Saturation1 : Saturate  UpperLimit=100000  LowerLimit=-100000
  Saturation2 : Saturate  UpperLimit=100000  LowerLimit=-100000
  Position : Outport
  wires:
  Saturation2/1 -> INT_Alt/1
  Saturation1/1 -> INT_Lon/1
  Saturation/1 -> INT_Lat/1
  Position_dot/1 -> Demux/1  "Position_dot"
  Demux/1 -> Saturation/1
  Demux/2 -> Saturation1/1
  Demux/3 -> Saturation2/1
  INT_Lat/1 -> Mux/1  "Lat"
  INT_Lon/1 -> Mux/2  "Lon"
  INT_Alt/1 -> Mux/3  "Alt"
  Mux/1 -> Position/1  "Position"

== system AircraftModel_6DoF/Equations of Motion/INT_vv_f ==
  vv_dot_f : Inport
  Demux : Demux  Outputs=3
  INT_u : Integrator  InitialCondition=TrimPoint.States.ubar  ContinuousStateAttributes='u'
  INT_v : Integrator  InitialCondition=TrimPoint.States.vbar  ContinuousStateAttributes='v'
  INT_w : Integrator  InitialCondition=TrimPoint.States.wbar  ContinuousStateAttributes='w'
  Mux : Mux  Inputs=3
  Saturation : Saturate  UpperLimit=100000  LowerLimit=-100000
  Saturation1 : Saturate  UpperLimit=100000  LowerLimit=-100000
  Saturation2 : Saturate  UpperLimit=100000  LowerLimit=-100000
  vv_f : Outport
  wires:
  vv_dot_f/1 -> Demux/1  "vv_dot_f"
  Demux/1 -> Saturation/1  "u_dot"
  Demux/2 -> Saturation1/1  "v_dot"
  Demux/3 -> Saturation2/1  "w_dot"
  INT_u/1 -> Mux/1  "u"
  INT_v/1 -> Mux/2  "v"
  INT_w/1 -> Mux/3  "w"
  Mux/1 -> vv_f/1  "vv_f"
  Saturation/1 -> INT_u/1
  Saturation1/1 -> INT_v/1
  Saturation2/1 -> INT_w/1

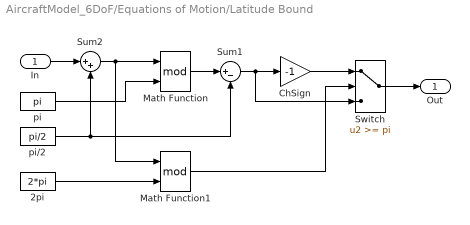
== system AircraftModel_6DoF/Equations of Motion/Latitude Bound ==
  In : Inport
  2pi : Constant  Value=2*pi  SampleTime=-1
  ChSign : Gain  Gain=-1  SaturateOnIntegerOverflow=on  OutDataTypeStr=Inherit: Same as input  ParamDataTypeStr=Inherit: Same as input
  Math Function : Math  Operator=mod  SignedPower=on  SaturateOnIntegerOverflow=on
  Math Function1 : Math  Operator=mod  SignedPower=on  SaturateOnIntegerOverflow=on
  Sum1 : Sum  Inputs=|+-  InputSameDT=on  SaturateOnIntegerOverflow=on  OutDataTypeStr=Inherit: Same as first input
  Sum2 : Sum  Inputs=|++  InputSameDT=on  SaturateOnIntegerOverflow=on  OutDataTypeStr=Inherit: Same as first input
  Switch : Switch  Threshold=pi  SaturateOnIntegerOverflow=on  InputSameDT=on
  pi : Constant  Value=pi  SampleTime=-1
  pi/2 : Constant  Value=pi/2  SampleTime=-1
  Out : Outport
  wires:
  pi/1 -> Math Function/2
  Math Function/1 -> Sum1/1
  pi/2/1 -> Sum1/2, Sum2/2
  Sum1/1 -> ChSign/1, Switch/3
  Math Function1/1 -> Switch/2
  Switch/1 -> Out/1
  In/1 -> Sum2/1
  Sum2/1 -> Math Function/1, Math Function1/1
  ChSign/1 -> Switch/1
  2pi/1 -> Math Function1/2

== system AircraftModel_6DoF/Equations of Motion/Longitude Bound ==
  In : Inport
  2pi : Constant  Value=2*pi  SampleTime=-1
  Math Function : Math  Operator=mod  SignedPower=on  SaturateOnIntegerOverflow=on
  Sum1 : Sum  Inputs=|+-  InputSameDT=on  SaturateOnIntegerOverflow=on  OutDataTypeStr=Inherit: Same as first input
  Sum2 : Sum  Inputs=|++  InputSameDT=on  SaturateOnIntegerOverflow=on  OutDataTypeStr=Inherit: Same as first input
  pi : Constant  Value=pi  SampleTime=-1
  Out : Outport
  wires:
  Sum1/1 -> Out/1
  pi/1 -> Sum1/2, Sum2/2
  Sum2/1 -> Math Function/1
  In/1 -> Sum2/1
  2pi/1 -> Math Function/2
  Math Function/1 -> Sum1/1

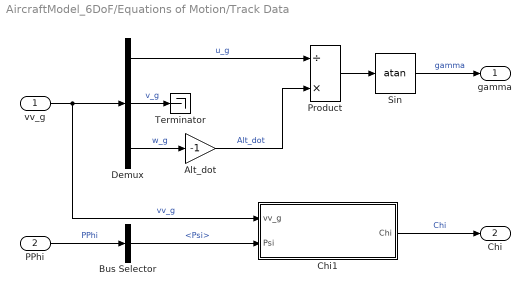
== system AircraftModel_6DoF/Equations of Motion/Track Data ==
  vv_g : Inport
  PPhi : Inport  Port=2  OutDataTypeStr=Bus: PPhi
  Alt_dot : Gain  Gain=-1
  Bus Selector : BusSelector  OutputSignals=Psi
  Chi1 : MATLAB Function  TreatAsAtomicUnit=on
  Demux : Demux  Outputs=3
  Product : Product  Inputs=/*
  Sin : Trigonometry  Operator=atan
  Terminator : Terminator
  gamma : Outport
  Chi : Outport  Port=2
  wires:
  Sin/1 -> gamma/1  "gamma"
  Demux/1 -> Product/1  "u_g"
  Product/1 -> Sin/1
  Demux/3 -> Alt_dot/1  "w_g"
  Alt_dot/1 -> Product/2  "Alt_dot"
  vv_g/1 -> Chi1/1(vv_g), Demux/1  "vv_g"
  Chi1/1(Chi) -> Chi/1  "Chi"
  Demux/2 -> Terminator/1  "v_g"
  PPhi/1 -> Bus Selector/1  "PPhi"
  Bus Selector/1 -> Chi1/2(Psi)  "<Psi>"

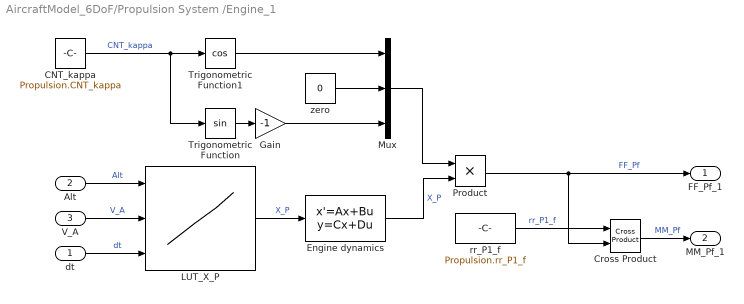
== system AircraftModel_6DoF/Propulsion System /Engine_1 ==
  dt : Inport
  Alt : Inport  Port=2
  V_A : Inport  Port=3
  CNT_kappa : Constant  Value=Propulsion.CNT_kappa  SampleTime=-1
  Cross Product : vrlib/Utilities/Cross Product
  Engine dynamics : StateSpace  A=Propulsion.Act_t.a  B=Propulsion.Act_t.b  C=Propulsion.Act_t.c  D=Propulsion.Act_t.d  InitialCondition=TrimPoint.States.X_P  ContinuousStateAttributes='X_P1'
  Gain : Gain  Gain=-1
  LUT_X_P : Lookup_n-D  NumberOfTableDimensions=3  BreakpointsForDimension1=Propulsion.LUT.LUT_Alt  BreakpointsForDimension2=Propulsion.LUT.LUT_V_A  BreakpointsForDimension3=Propulsion.LUT.LUT_dt  Table=Propulsion.LUT.LUT_X_P  ExtrapMethod=Clip  InputSameDT=on
      settings: InputPortMap=u0,u1,u2
  Mux : Mux  Inputs=3
  Product : Product  RndMeth=Zero
  Trigonometric Function : Trigonometry
  Trigonometric Function1 : Trigonometry  Operator=cos
  "rr_P1_f " : Constant  Value=Propulsion.rr_P1_f  SampleTime=-1
  zero : Constant  Value=0  SampleTime=-1
  FF_Pf_1 : Outport
  MM_Pf_1 : Outport  Port=2
  wires:
  Alt/1 -> LUT_X_P/1  "Alt"
  V_A/1 -> LUT_X_P/2  "V_A"
  dt/1 -> LUT_X_P/3  "dt"
  zero/1 -> Mux/2
  Mux/1 -> Product/1
  Engine dynamics/1 -> Product/2  "X_P"
  CNT_kappa/1 -> Trigonometric Function1/1, Trigonometric Function/1  "CNT_kappa"
  Trigonometric Function1/1 -> Mux/1
  Product/1 -> FF_Pf_1/1, Cross Product/2  "FF_Pf"
  Cross Product/1 -> MM_Pf_1/1  "MM_Pf"
  Trigonometric Function/1 -> Gain/1
  Gain/1 -> Mux/3
  LUT_X_P/1 -> Engine dynamics/1  "X_P"
  "rr_P1_f "/1 -> Cross Product/1  "rr_P1_f"

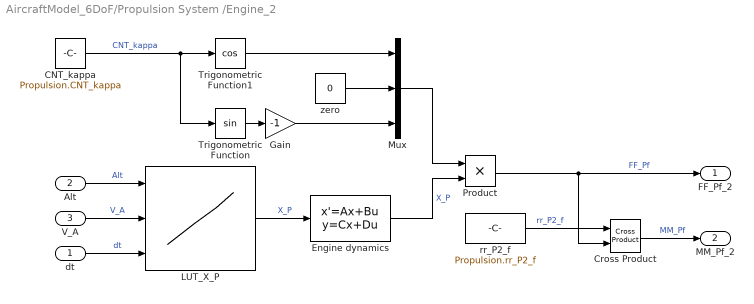
== system AircraftModel_6DoF/Propulsion System /Engine_2 ==
  dt : Inport
  Alt : Inport  Port=2
  V_A : Inport  Port=3
  CNT_kappa : Constant  Value=Propulsion.CNT_kappa  SampleTime=-1
  Cross Product : vrlib/Utilities/Cross Product
  Engine dynamics : StateSpace  A=Propulsion.Act_t.a  B=Propulsion.Act_t.b  C=Propulsion.Act_t.c  D=Propulsion.Act_t.d  InitialCondition=TrimPoint.States.X_P  ContinuousStateAttributes='X_P2'
  Gain : Gain  Gain=-1
  LUT_X_P : Lookup_n-D  NumberOfTableDimensions=3  BreakpointsForDimension1=Propulsion.LUT.LUT_Alt  BreakpointsForDimension2=Propulsion.LUT.LUT_V_A  BreakpointsForDimension3=Propulsion.LUT.LUT_dt  Table=Propulsion.LUT.LUT_X_P  ExtrapMethod=Clip  InputSameDT=on
      settings: InputPortMap=u0,u1,u2
  Mux : Mux  Inputs=3
  Product : Product  RndMeth=Zero
  Trigonometric Function : Trigonometry
  Trigonometric Function1 : Trigonometry  Operator=cos
  "rr_P2_f " : Constant  Value=Propulsion.rr_P2_f  SampleTime=-1
  zero : Constant  Value=0  SampleTime=-1
  FF_Pf_2 : Outport
  MM_Pf_2 : Outport  Port=2
  wires:
  zero/1 -> Mux/2
  Gain/1 -> Mux/3
  Mux/1 -> Product/1
  Cross Product/1 -> MM_Pf_2/1  "MM_Pf"
  Trigonometric Function1/1 -> Mux/1
  Product/1 -> FF_Pf_2/1, Cross Product/2  "FF_Pf"
  Trigonometric Function/1 -> Gain/1
  Alt/1 -> LUT_X_P/1  "Alt"
  dt/1 -> LUT_X_P/3  "dt"
  LUT_X_P/1 -> Engine dynamics/1  "X_P"
  V_A/1 -> LUT_X_P/2  "V_A"
  "rr_P2_f "/1 -> Cross Product/1  "rr_P2_f"
  CNT_kappa/1 -> Trigonometric Function1/1, Trigonometric Function/1  "CNT_kappa"
  Engine dynamics/1 -> Product/2  "X_P"

== system AircraftModel_6DoF/Equations of Motion/Calculation of Position_dot/ZeroOffset - cos (Lat) ==
  In : Inport
  Abs : Abs  SaturateOnIntegerOverflow=on
  Constant : Constant  Value=tol  SampleTime=-1
  Non-zero Sign : Subsystem  mask(Non-zero sign){}
      mask help: Sign function outputs 1 for input greater than or equal to 0, and -1 otherwise.
  Product : Product  InputSameDT=on  SaturateOnIntegerOverflow=on  OutDataTypeStr=Inherit: Same as first input
  Switch : Switch  Threshold=tol  SaturateOnIntegerOverflow=on  InputSameDT=on
  Out : Outport
  wires:
  In/1 -> Switch/1, Non-zero Sign/1(In), Abs/1
  Abs/1 -> Switch/2
  Non-zero Sign/1(Out) -> Product/1
  Constant/1 -> Product/2
  Product/1 -> Switch/3
  Switch/1 -> Out/1

== system AircraftModel_6DoF/Equations of Motion/Calculation of Position_dot/ZeroOffset - cos (Lat)/Non-zero Sign ==
  In : Inport
  One : Constant  SampleTime=-1
  Relational Operator : RelationalOperator  Operator===  RndMeth=Nearest  InputSameDT=on
  Sign : Signum
  Switch : Switch  Threshold=1  SaturateOnIntegerOverflow=on  InputSameDT=on
  Zero : Constant  Value=0  SampleTime=-1
  Out : Outport
  wires:
  Zero/1 -> Relational Operator/2
  In/1 -> Relational Operator/1, Sign/1
  Relational Operator/1 -> Switch/2
  One/1 -> Switch/1
  Sign/1 -> Switch/3
  Switch/1 -> Out/1

== matlab function AircraftModel_6DoF/Equations of Motion/Track Data/Chi1 ==
  data: vv_g input size=3; Chi output; Psi input
%%%%%%%%%%%%%%%%%%%%%%%%%%%%%
% Calculation of Track Data %
%%%%%%%%%%%%%%%%%%%%%%%%%%%%%

function Chi  = fcn(vv_g,Psi)

u_g = vv_g(1);
v_g = vv_g(2);

if abs(u_g)>1E-5 && abs(v_g)>1E-5
    Chi_pi_Bound = atan2(v_g,u_g);
else
    Chi_pi_Bound = Psi;
end
Chi = mod(Chi_pi_Bound,2*pi);

== matlab function AircraftModel_6DoF/Equations of Motion/Calculation of Position_dot/WGS84 ==
  data: CNT_a input; CNT_f input; Lat input; R_M output; R_N output
%%%%%%%%%%%%%%%%%%%
% WGS84 ellipsoid %
%%%%%%%%%%%%%%%%%%%

% ref: National Imagery And Mapping Agency (NIMA): Department of Defense World Geodetic System 1984. Third Edition. NIMA, 2000 - TR8350.2 

function [R_M, R_N] = fcn(CNT_a, CNT_f, Lat)

%-------------------------------------------------------------------------%
% first eccentricity
CNT_epsilon = sqrt(CNT_f*(2-CNT_f));
% meridian radius
R_M = (CNT_a*(1-CNT_epsilon^2))/(1-CNT_epsilon^2*sin(Lat)^2)^(3/2);
% normal radius
R_N = CNT_a/sqrt(1-CNT_epsilon^2*sin(Lat)^2);

== matlab function AircraftModel_6DoF/Equations of Motion/PPhi Calculation ==
  data: CC_gf output; CC_fg output size=[3 3]; PPhi output size=3; PPhi_In input size=3
function [CC_gf,CC_fg,PPhi] = fcn(PPhi_In)

Phi = mod(PPhi_In(1)+pi,2*pi)-pi; % pi bound
Theta = mod(PPhi_In(2)+pi,2*pi)-pi; % pi bound
Psi = mod(PPhi_In(3)+pi,2*pi)-pi; % pi bound
% Psi_2pi = mod(PPhi_In(3),2*pi); % 2pi bound

PPhi = [Phi; Theta; Psi];

CC_fg = [cos(Psi)*cos(Theta)                                        sin(Psi)*cos(Theta)                         -sin(Theta);
         cos(Psi)*sin(Theta)*sin(Phi)-sin(Psi)*cos(Phi) sin(Psi)*sin(Theta)*sin(Phi)+cos(Psi)*cos(Phi)  cos(Theta)*sin(Phi);
         cos(Psi)*sin(Theta)*cos(Phi)+sin(Psi)*sin(Phi) sin(Psi)*sin(Theta)*cos(Phi)-cos(Psi)*sin(Phi)  cos(Theta)*cos(Phi)];
     
CC_gf = CC_fg';

== matlab function AircraftModel_6DoF/Equations of Motion/PPhi_dot Calculation ==
  data: OOmega_f input; PPhi_dot output; PPhi input
%%%%%%%%%%%%%%%%%%%%%%%%%%%
% Calculation of PPhi_dot %
%%%%%%%%%%%%%%%%%%%%%%%%%%%

function PPhi_dot = fcn(OOmega_f,PPhi)

if cos(PPhi(2))<1E-5
    PPhi_dot = [0 0 0]';
else
    PPhi_dot = [1 sin(PPhi(1))*tan(PPhi(2))  cos(PPhi(1))*tan(PPhi(2)); ...
                0 cos(PPhi(1))              -sin(PPhi(1))             ; ...
                0 sin(PPhi(1))/cos(PPhi(2))  cos(PPhi(1))/cos(PPhi(2))]*OOmega_f;
end

== matlab function AircraftModel_6DoF/Aerodynamics/X_A ==
  data: S input; AirData input Bus: AirData size=1; C_X0 input; C_Xa input; C_Xa2 input; C_Xb2 input; X_A output

%%%%%%%%%%%%%%%%%%%%%%
% Body-fixed X force %
%%%%%%%%%%%%%%%%%%%%%%

function X_A = fcn(S,AirData,C_X0,C_Xa,C_Xa2,C_Xb2)

X_A = AirData.p_dyn*S*(C_X0 + ...
                           C_Xa*AirData.alpha + ...
                           C_Xa2*(AirData.alpha)^2 + ...
                           C_Xb2*(AirData.beta)^2);

== matlab function AircraftModel_6DoF/Aerodynamics/Y_A ==
  data: S input; cbar input; AirData input Bus: AirData size=1; Act input; OOmega_f input; C_Yb input; C_Yp input; C_Yr input; C_Ydr input; Y_A output

%%%%%%%%%%%%%%%%%%%%%%
% Body-fixed Y force %
%%%%%%%%%%%%%%%%%%%%%%

function Y_A = fcn(S,cbar,AirData,Act,OOmega_f,C_Yb,C_Yp,C_Yr,C_Ydr)

Y_A = AirData.p_dyn*S*(C_Yb*AirData.beta + ...
                           C_Yp*OOmega_f.p*cbar/AirData.V_A + ...
                           C_Yr*OOmega_f.r*cbar/AirData.V_A + ...
                           C_Ydr*Act.dr);

== matlab function AircraftModel_6DoF/Aerodynamics/Z_A ==
  data: S input; cbar input; AirData input Bus: AirData size=1; Act input; OOmega_f input; C_Z0 input; C_Za input; C_Zq input; C_Zde input; Z_A output

%%%%%%%%%%%%%%%%%%%%%%
% Body-fixed Z force %
%%%%%%%%%%%%%%%%%%%%%%

function Z_A = fcn(S,cbar,AirData,Act,OOmega_f,C_Z0,C_Za,C_Zq,C_Zde)

Z_A = AirData.p_dyn*S*(C_Z0 + ...
                           C_Za*AirData.alpha + ...
                           C_Zq*OOmega_f.q*cbar/AirData.V_A + ...
                           C_Zde*Act.de);

== matlab function AircraftModel_6DoF/Aerodynamics/L_A ==
  data: S input; cbar input; AirData input Bus: AirData size=1; Act input; OOmega_f input; C_lb input; C_lp input; C_lr input; C_lda input; C_ldr input; L_A output

%%%%%%%%%%%%%%%%%%%%%%%%%%
% Body-fixed roll moment %
%%%%%%%%%%%%%%%%%%%%%%%%%%

function L_A = fcn(S,cbar,AirData,Act,OOmega_f,C_lb,C_lp,C_lr,C_lda,C_ldr)

L_A = AirData.p_dyn*S*cbar*(C_lb*AirData.beta + ...
                                    C_lp*OOmega_f.p*cbar/AirData.V_A + ...
                                    C_lr*OOmega_f.r*cbar/AirData.V_A + ...
                                    C_lda*Act.da + ...
                                    C_ldr*Act.dr);

== matlab function AircraftModel_6DoF/Aerodynamics/M_A ==
  data: S input; cbar input; AirData input Bus: AirData size=1; Act input; OOmega_f input; C_m0 input; C_ma input; C_mq input; C_mde input; M_A output

%%%%%%%%%%%%%%%%%%%%%%%%%%%
% Body-fixed pitch moment %
%%%%%%%%%%%%%%%%%%%%%%%%%%%

function M_A = fcn(S,cbar,AirData,Act,OOmega_f,C_m0,C_ma,C_mq,C_mde)

M_A = AirData.p_dyn*S*cbar*(C_m0 + ...
                                    C_ma*AirData.alpha + ...
                                    C_mq*OOmega_f.q*cbar/AirData.V_A + ...
                                    C_mde*Act.de);

== matlab function AircraftModel_6DoF/Aerodynamics/N_A ==
  data: S input; cbar input; AirData input Bus: AirData size=1; Act input; OOmega_f input; C_nb input; C_np input; C_nr input; C_nda input; C_ndr input; N_A output

%%%%%%%%%%%%%%%%%%%%%%%%%
% Body-fixed yaw moment %
%%%%%%%%%%%%%%%%%%%%%%%%%

function N_A = fcn(S,cbar,AirData,Act,OOmega_f,C_nb,C_np,C_nr,C_nda,C_ndr)

N_A = AirData.p_dyn*S*cbar*(C_nb*AirData.beta + ...
                                    C_np*OOmega_f.p*cbar/AirData.V_A + ...
                                    C_nr*OOmega_f.r*cbar/AirData.V_A + ...
                                    C_nda*Act.da + ...
                                    C_ndr*Act.dr);
